simulink model "hw2_p8_a"  (R2020a)
settings: Solver=VariableStepAuto  StartTime=0.0  StopTime=60  RelTol=1e-7
settings Model: Creator=Tomo  LastModifiedBy=Tomo

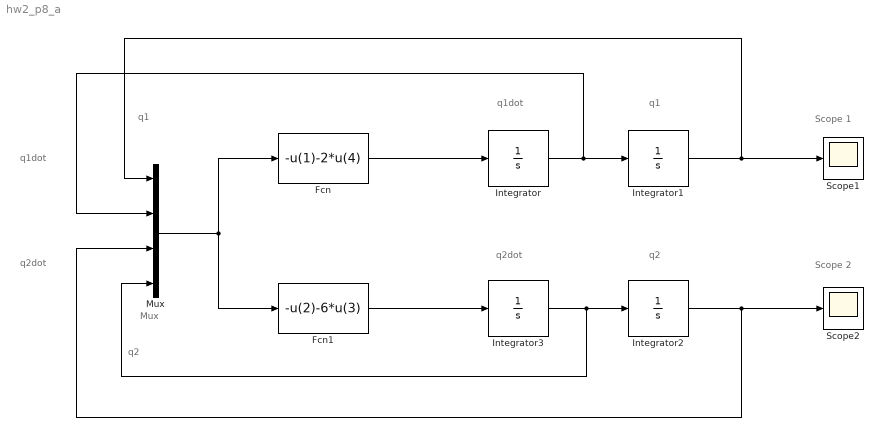
== system hw2_p8_a ==
  note: Scope 1
  note: q1dot
  note: q2dot
  note: q1
  note: q2
  note: q1
  note: q1dot
  note: q2
  note: q2dot
  note: Mux
  note: Scope 2
  Fcn : Fcn  Expr=-u(1)-2*u(4)
  Fcn1 : Fcn  Expr=-u(2)-6*u(3)
  Integrator : Integrator
  Integrator1 : Integrator  InitialCondition=2
  Integrator2 : Integrator
  Integrator3 : Integrator
  Mux : Mux
  Scope1 : Scope
  Scope2 : Scope
  wires:
  Mux/1 -> Fcn1/1, Fcn/1
  Fcn/1 -> Integrator/1
  Integrator/1 -> Mux/2, Integrator1/1
  Integrator1/1 -> Mux/1, Scope1/1
  Fcn1/1 -> Integrator3/1
  Integrator3/1 -> Mux/4, Integrator2/1
  Integrator2/1 -> Mux/3, Scope2/1
